simulink model "model3"  (R2024b)
settings: Solver=VariableStepAuto  StartTime=0.0  StopTime=10.0  RelTol=1e-3
settings Model: Creator=muradaliyev  LastModifiedBy=muradaliyev

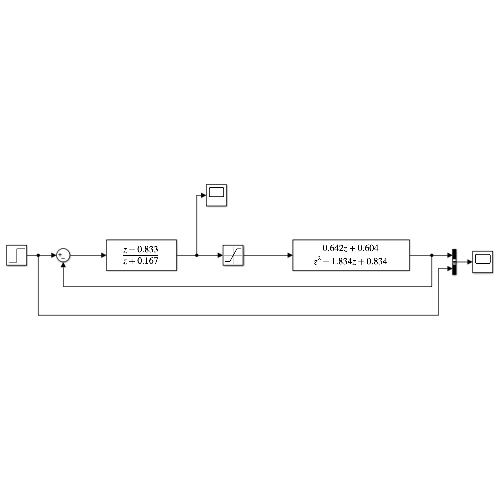
[thumbnail: Simulink's stored preview of the top-level diagram]
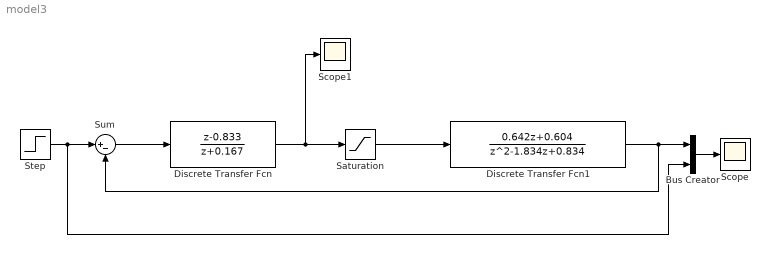
== system model3 ==
  Bus Creator : BusCreator  Inputs=2
  Discrete Transfer Fcn : DiscreteTransferFcn  Numerator=[1 -0.833]  Denominator=[1 0.167]
  Discrete Transfer Fcn1 : DiscreteTransferFcn  Numerator=[0.642 0.604]  Denominator=[1 -1.834 0.834]
  Saturation : Saturate
  Scope : Scope
  Scope1 : Scope
  Step : Step  SampleTime=0.1
  Sum : Sum  Inputs=|+-
  wires:
  Sum/1 -> Discrete Transfer Fcn/1
  Step/1 -> Bus Creator/2, Sum/1
  Bus Creator/1 -> Scope/1
  Discrete Transfer Fcn1/1 -> Sum/2, Bus Creator/1
  Saturation/1 -> Discrete Transfer Fcn1/1
  Discrete Transfer Fcn/1 -> Scope1/1, Saturation/1
